simulink model "lqr_nao_linear_simulink"  (R2022a)
settings: Solver=VariableStepAuto  StartTime=0  StopTime=200  RelTol=1e-3
values from neighbouring files (symbols this model uses):
  A = [ 0 1 0  0 ... (first row only)    [ball_and_beam_pfc.m]
  amplitude_entrada = 1    [ball_and_beam_pfc.m]
  B = [0 ... (first row only)    [ball_and_beam_pfc.m]
  bool_degrau = 1    [ball_and_beam_pfc.m]
  C = [0 0 1 0]    [ball_and_beam_pfc.m]
  g = 9.8    [ball_and_beam_pfc.m]    (also in nonlinear_ball_and_beam.m)
  Jv = (1/2) * mv * L^2    (= 0.058703125)    [ball_and_beam_pfc.m]    (also in nonlinear_ball_and_beam.m)
  k_seguimento_lqr = K_nulo(1:4)    [ball_and_beam_pfc.m]
  ki_seguimento_lqr = K_nulo(5)    [ball_and_beam_pfc.m]
  L = 0.425    [ball_and_beam_pfc.m]    (also in nonlinear_ball_and_beam.m)
  L_observador = inv(T)*Lchp    [ball_and_beam_pfc.m]
  mb = 0.064    [ball_and_beam_pfc.m]    (also in nonlinear_ball_and_beam.m)
  mv = 0.65    [ball_and_beam_pfc.m]    (also in nonlinear_ball_and_beam.m)
libraries: mpclib x1
settings Model: Creator=Notebook_Artur  LastModifiedBy=Notebook_Artur

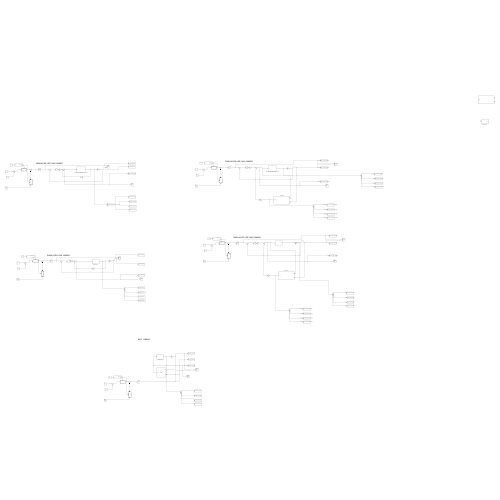
[thumbnail: Simulink's stored preview of the top-level diagram]
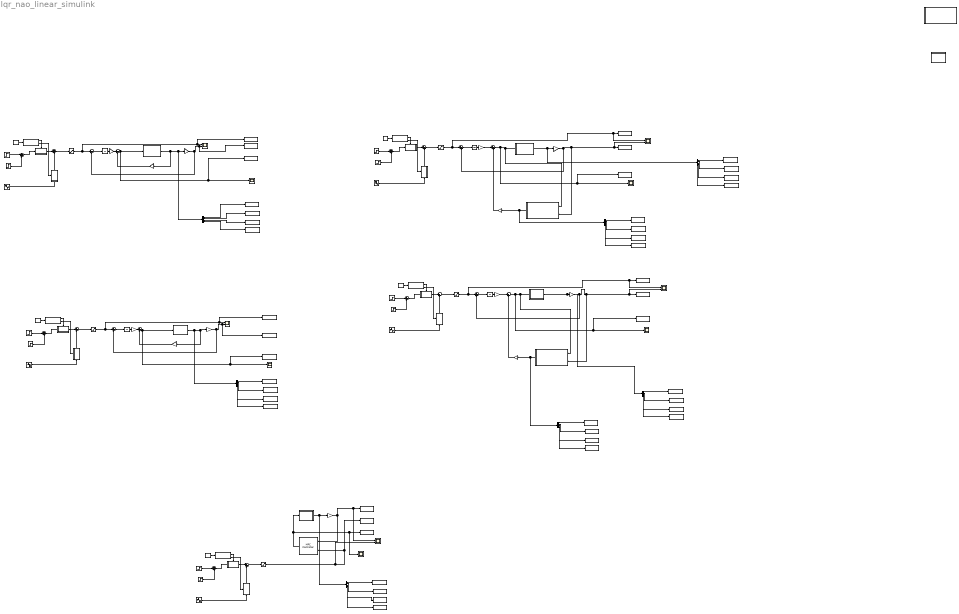
== system lqr_nao_linear_simulink ==
  note: SIMULAÇÃO LQR NAO LINEAR ENTRADA NORMAL
  note: SIMULAÇÃO LQR LINEAR ENTRADA NORMAL
  note: SIMULAÇÃO LQR NAO LINEAR ENTRADA NORMAL
  note: SIMULAÇÃO LQR NAO LINEAR ENTRADA NORMAL
  note: MPC LINEAR
  Constant{1..5} (5 alike) : Constant  Value=bool_degrau
  Demux{,1..6} (7 alike) : Demux
  Gain{1,4,7,29} (4 alike) : Gain  Gain=k_seguimento_lqr  Multiplication=Matrix(K*u)
  Gain{2,5,8,30,54} (5 alike) : Gain  Gain=C  Multiplication=Matrix(K*u)
  Gain{3,6,9,31} (4 alike) : Gain  Gain=ki_seguimento_lqr
  If{,1..4} (5 alike) : If  IfExpression=u1 == 1
  If Action Subsystem1 : Subsystem  TreatAsAtomicUnit=on
  If Action Subsystem10 : Subsystem  TreatAsAtomicUnit=on
  If Action Subsystem2 : Subsystem  TreatAsAtomicUnit=on
  If Action Subsystem3 : Subsystem  TreatAsAtomicUnit=on
  If Action Subsystem4 : Subsystem  TreatAsAtomicUnit=on
  If Action Subsystem5 : Subsystem  TreatAsAtomicUnit=on
  If Action Subsystem6 : Subsystem  TreatAsAtomicUnit=on
  If Action Subsystem7 : Subsystem  TreatAsAtomicUnit=on
  If Action Subsystem8 : Subsystem  TreatAsAtomicUnit=on
  If Action Subsystem9 : Subsystem  TreatAsAtomicUnit=on
  Integrator{1..3,5} (4 alike) : Integrator
  MPC Controller1 : mpclib/MPC Controller  SCDEnableBlockLinearizationSpecification=on  mpcobj=mpc1  is_multiple=0  enable_value=0  return_u0=off  updateMPCinCallerWorkspace=on  md_inport=off  mv_inport=off  uref_inport=off  return_cost=off  return_mvseq=off  return_qpstatus=off  return_xseq=off  return_state=off  return_ovseq=off  state_inport=off  umin_inport=off  umax_inport=off  ymin_inport=off  ymax_inport=off  cc_inport=off  ywt_inport=off  uwt_inport=off  duwt_inport=off  rhoeps_inport=off  pm_inport=off  MaximumP=10  HorizonChoice=FixedHorizon  n_ts=0.1  n_p=10  n_mv=1  n_md=0  n_ud=0  n_mo=1  n_uo=0  BlockDataType=double  SampleTimeInherited=off  switch_inport=off
  Modelo Linear : Subsystem
  Modelo Linear1 : Subsystem
  Modelo Linear2 : Subsystem
  Modelo Linear3 : Subsystem
  Modelo ball and beam nao linear - Final : Subsystem
  Modelo ball and beam nao linear - Final1 : Subsystem
  Observador1 : Subsystem
  Observador2 : Subsystem
  Observador3 : Subsystem
  Saturation{,1..4} (5 alike) : Saturate  UpperLimit=L/2  LowerLimit=-L/2
  Scope{,2..3,5,8} (5 alike) : Scope
  Scope{1,4,6..7,13} (5 alike) : Scope  NumInputPorts=2
  Sine Wave{1..5} (5 alike) : Sin  Amplitude=amplitude_entrada  Frequency=0.1  SampleTime=0
  Step{1,3,5..6,8} (5 alike) : Step  After=amplitude_entrada  SampleTime=0
  Step{2,4,7,9..10} (5 alike) : Step  Time=100  After=-2*amplitude_entrada  SampleTime=0
  Sum{,1,4..5,8..9,12..14,20} (10 alike) : Sum  Inputs=|++
  Sum{2..3,6..7,10..11,15..16} (8 alike) : Sum  Inputs=|+-
  To Workspace : ToWorkspace  VariableName=y_output_nao_linear  SaveFormat=Timeseries  SampleTime=-1
  To Workspace1 : ToWorkspace  VariableName=u_output_nao_linear  SaveFormat=Timeseries  SampleTime=-1
  To Workspace10 : ToWorkspace  VariableName=y_output_nao_linear_observador  SaveFormat=Timeseries  SampleTime=-1
  To Workspace11 : ToWorkspace  VariableName=u_output_nao_linear_observador  SaveFormat=Timeseries  SampleTime=-1
  To Workspace12 : ToWorkspace  VariableName=acao_controle_nao_linear_observador  SaveFormat=Timeseries  SampleTime=-1
  To Workspace13 : ToWorkspace  VariableName=estados_nao_linear_estimados_observador2  SaveFormat=Timeseries  SampleTime=-1
  To Workspace14 : ToWorkspace  VariableName=estados_linear1  SaveFormat=Timeseries  SampleTime=-1
  To Workspace15 : ToWorkspace  VariableName=estados_linear_observador1  SaveFormat=Timeseries  SampleTime=-1
  To Workspace16 : ToWorkspace  VariableName=estados_linear2  SaveFormat=Timeseries  SampleTime=-1
  To Workspace17 : ToWorkspace  VariableName=estados_linear3  SaveFormat=Timeseries  SampleTime=-1
  To Workspace18 : ToWorkspace  VariableName=estados_linear4  SaveFormat=Timeseries  SampleTime=-1
  To Workspace19 : ToWorkspace  VariableName=estados_nao_linear1  SaveFormat=Timeseries  SampleTime=-1
  To Workspace2 : ToWorkspace  VariableName=y_output_linear  SaveFormat=Timeseries  SampleTime=-1
  To Workspace20 : ToWorkspace  VariableName=estados_nao_linear2  SaveFormat=Timeseries  SampleTime=-1
  To Workspace21 : ToWorkspace  VariableName=estados_nao_linear3  SaveFormat=Timeseries  SampleTime=-1
  To Workspace22 : ToWorkspace  VariableName=estados_nao_linear4  SaveFormat=Timeseries  SampleTime=-1
  To Workspace23 : ToWorkspace  VariableName=estados_linear_observador2  SaveFormat=Timeseries  SampleTime=-1
  To Workspace24 : ToWorkspace  VariableName=estados_linear_observador3  SaveFormat=Timeseries  SampleTime=-1
  To Workspace25 : ToWorkspace  VariableName=estados_linear_observador4  SaveFormat=Timeseries  SampleTime=-1
  To Workspace26 : ToWorkspace  VariableName=estados_linear_estimados_observador1  SaveFormat=Timeseries  SampleTime=-1
  To Workspace27 : ToWorkspace  VariableName=estados_linear_estimados_observador2  SaveFormat=Timeseries  SampleTime=-1
  To Workspace28 : ToWorkspace  VariableName=estados_linear_estimados_observador3  SaveFormat=Timeseries  SampleTime=-1
  To Workspace29 : ToWorkspace  VariableName=estados_linear_estimados_observador4  SaveFormat=Timeseries  SampleTime=-1
  To Workspace3 : ToWorkspace  VariableName=u_output_linear  SaveFormat=Timeseries  SampleTime=-1
  To Workspace30 : ToWorkspace  VariableName=estados_nao_linear_estimados_observador3  SaveFormat=Timeseries  SampleTime=-1
  To Workspace31 : ToWorkspace  VariableName=estados_nao_linear_estimados_observador4  SaveFormat=Timeseries  SampleTime=-1
  To Workspace32 : ToWorkspace  VariableName=estados_nao_linear_observador1  SaveFormat=Timeseries  SampleTime=-1
  To Workspace33 : ToWorkspace  VariableName=estados_nao_linear_observador2  SaveFormat=Timeseries  SampleTime=-1
  To Workspace34 : ToWorkspace  VariableName=estados_nao_linear_observador3  SaveFormat=Timeseries  SampleTime=-1
  To Workspace35 : ToWorkspace  VariableName=estados_nao_linear_observador4  SaveFormat=Timeseries  SampleTime=-1
  To Workspace36 : ToWorkspace  VariableName=estados_mpc_linear1  SaveFormat=Timeseries  SampleTime=-1
  To Workspace37 : ToWorkspace  VariableName=estados_mpc_linear2  SaveFormat=Timeseries  SampleTime=-1
  To Workspace38 : ToWorkspace  VariableName=estados_mpc_linear3  SaveFormat=Timeseries  SampleTime=-1
  To Workspace39 : ToWorkspace  VariableName=estados_mpc_linear4  SaveFormat=Timeseries  SampleTime=-1
  To Workspace4 : ToWorkspace  VariableName=acao_controle_linear  SaveFormat=Timeseries  SampleTime=-1
  To Workspace40 : ToWorkspace  VariableName=y_output_mpc_linear  SaveFormat=Timeseries  SampleTime=-1
  To Workspace41 : ToWorkspace  VariableName=acao_controle_mpc_linear  SaveFormat=Timeseries  SampleTime=-1
  To Workspace42 : ToWorkspace  VariableName=u_output_mpc_linear  SaveFormat=Timeseries  SampleTime=-1
  To Workspace5 : ToWorkspace  VariableName=acao_controle_nao_linear  SaveFormat=Timeseries  SampleTime=-1
  To Workspace6 : ToWorkspace  VariableName=y_output_linear_observador  SaveFormat=Timeseries  SampleTime=-1
  To Workspace7 : ToWorkspace  VariableName=u_output_linear_observador  SaveFormat=Timeseries  SampleTime=-1
  To Workspace8 : ToWorkspace  VariableName=acao_controle_linear_observador  SaveFormat=Timeseries  SampleTime=-1
  To Workspace9 : ToWorkspace  VariableName=estados_nao_linear_estimados_observador1  SaveFormat=Timeseries  SampleTime=-1
  wires:
  Sum16/1 -> Integrator5/1
  Gain30/1 -> Sum16/2, To Workspace/1, Scope13/2
  Step9/1 -> Sum20/2
  Gain29/1 -> Sum15/2
  Step6/1 -> Sum20/1
  Gain31/1 -> Sum15/1
  Integrator5/1 -> Gain31/1
  Saturation/1 -> To Workspace1/1, Scope13/1, Sum16/1
  Sine Wave1/1 -> If Action Subsystem1/1(In1)
  If Action Subsystem1/1(Out1) -> Sum/2
  Sum20/1 -> If Action Subsystem2/1(In1)
  If Action Subsystem2/1(Out1) -> Sum/1
  Sum/1 -> Saturation/1
  Constant2/1 -> If/1
  If/1 -> If Action Subsystem2/Action
  If/2 -> If Action Subsystem1/Action
  Sum15/1 -> Modelo ball and beam nao linear - Final/1(In1), To Workspace5/1, Scope2/1
  If1/1 -> If Action Subsystem4/Action
  If Action Subsystem3/1(Out1) -> Sum1/2
  Sum1/1 -> Saturation1/1
  If Action Subsystem4/1(Out1) -> Sum1/1
  If1/2 -> If Action Subsystem3/Action
  Integrator1/1 -> Gain3/1
  Gain3/1 -> Sum2/1
  Step1/1 -> Sum4/1
  Sine Wave2/1 -> If Action Subsystem3/1(In1)
  Sum2/1 -> Modelo Linear1/1(Input), To Workspace4/1, Scope3/1
  Gain1/1 -> Sum2/2
  Saturation1/1 -> To Workspace3/1, Scope1/1, Sum3/1
  Sum3/1 -> Integrator1/1
  Sum4/1 -> If Action Subsystem4/1(In1)
  Gain2/1 -> Sum3/2, To Workspace2/1, Scope1/2
  Step2/1 -> Sum4/2
  Constant1/1 -> If1/1
  Constant3/1 -> If2/1
  Modelo Linear2/1(Output) -> Demux2/1, Gain5/1
  If2/1 -> If Action Subsystem6/Action
  Gain4/1 -> Sum6/2
  Step4/1 -> Sum8/2
  Sum6/1 -> To Workspace8/1, Scope5/1, Observador1/1(ref), Modelo Linear2/1(Input)
  Sum7/1 -> Integrator2/1
  Gain5/1 -> Sum7/2, Scope4/2, To Workspace6/1, Observador1/2(y)
  Saturation2/1 -> To Workspace7/1, Scope4/1, Sum7/1
  Step3/1 -> Sum8/1
  Gain6/1 -> Sum6/1
  If Action Subsystem6/1(Out1) -> Sum5/1
  Sum5/1 -> Saturation2/1
  Integrator2/1 -> Gain6/1
  If2/2 -> If Action Subsystem5/Action
  Sine Wave3/1 -> If Action Subsystem5/1(In1)
  Sum8/1 -> If Action Subsystem6/1(In1)
  If Action Subsystem5/1(Out1) -> Sum5/2
  Observador1/1(x_chp) -> Demux3/1, Gain4/1
  If Action Subsystem7/1(Out1) -> Sum9/2
  If Action Subsystem8/1(Out1) -> Sum9/1
  If3/2 -> If Action Subsystem7/Action
  Gain9/1 -> Sum10/1
  Step5/1 -> Sum12/1
  Sine Wave4/1 -> If Action Subsystem7/1(In1)
  Integrator3/1 -> Gain9/1
  Sum12/1 -> If Action Subsystem8/1(In1)
  Saturation3/1 -> To Workspace11/1, Scope7/1, Sum11/1
  Sum9/1 -> Saturation3/1
  Gain8/1 -> Scope7/2, To Workspace10/1, Observador3/2(y), Sum11/2
  Constant4/1 -> If3/1
  Gain7/1 -> Sum10/2
  Sum10/1 -> To Workspace12/1, Scope8/1, Observador3/1(ref), Modelo ball and beam nao linear - Final1/1(In1)
  If3/1 -> If Action Subsystem8/Action
  Observador3/1(x_chp) -> Demux4/1, Gain7/1
  Step7/1 -> Sum12/2
  Sum11/1 -> Integrator3/1
  Modelo ball and beam nao linear - Final1/1(Out1) -> Demux5/1, Gain8/1
  Modelo Linear1/1(Output) -> Demux/1, Gain2/1, Gain1/1
  Modelo ball and beam nao linear - Final/1(Out1) -> Demux1/1, Gain30/1, Gain29/1
  Demux/1 -> To Workspace14/1
  Demux/2 -> To Workspace16/1
  Demux/3 -> To Workspace17/1
  Demux/4 -> To Workspace18/1
  Demux1/3 -> To Workspace21/1
  Demux1/4 -> To Workspace22/1
  Demux1/2 -> To Workspace20/1
  Demux1/1 -> To Workspace19/1
  Demux2/3 -> To Workspace24/1
  Demux2/4 -> To Workspace25/1
  Demux2/2 -> To Workspace23/1
  Demux2/1 -> To Workspace15/1
  Demux3/1 -> To Workspace26/1
  Demux3/4 -> To Workspace29/1
  Demux3/3 -> To Workspace28/1
  Demux3/2 -> To Workspace27/1
  Demux4/1 -> To Workspace9/1
  Demux4/4 -> To Workspace31/1
  Demux4/2 -> To Workspace13/1
  Demux4/3 -> To Workspace30/1
  Demux5/1 -> To Workspace32/1
  Demux5/4 -> To Workspace35/1
  Demux5/3 -> To Workspace34/1
  Demux5/2 -> To Workspace33/1
  Sine Wave5/1 -> If Action Subsystem9/1(In1)
  Sum14/1 -> If Action Subsystem10/1(In1)
  If4/2 -> If Action Subsystem9/Action
  Sum13/1 -> Saturation4/1
  If Action Subsystem10/1(Out1) -> Sum13/1
  Step8/1 -> Sum14/1
  If Action Subsystem9/1(Out1) -> Sum13/2
  Step10/1 -> Sum14/2
  Constant5/1 -> If4/1
  If4/1 -> If Action Subsystem10/Action
  MPC Controller1/1 -> Modelo Linear3/1(Input), Scope/1, To Workspace41/1
  Gain54/1 -> Scope6/1, To Workspace40/1, MPC Controller1/1
  Saturation4/1 -> Scope6/2, MPC Controller1/2, To Workspace42/1
  Demux6/4 -> To Workspace39/1
  Demux6/1 -> To Workspace36/1
  Demux6/3 -> To Workspace38/1
  Demux6/2 -> To Workspace37/1
  Modelo Linear3/1(Output) -> Demux6/1, Gain54/1

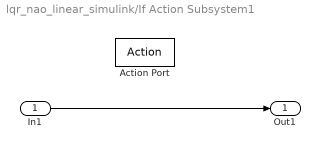
== system lqr_nao_linear_simulink/If Action Subsystem1 ==
  In1 : Inport
  Action Port : ActionPort  ActionPortLabel=else
  Out1 : Outport
  wires:
  In1/1 -> Out1/1

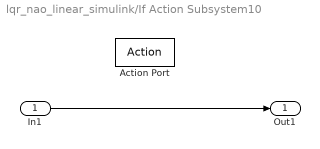
== system lqr_nao_linear_simulink/If Action Subsystem10 ==
  In1 : Inport
  Action Port : ActionPort  ActionPortLabel=if(u1 == 1)
  Out1 : Outport
  wires:
  In1/1 -> Out1/1

== system lqr_nao_linear_simulink/If Action Subsystem2 ==
  In1 : Inport
  Action Port : ActionPort  ActionPortLabel=if(u1 == 1)
  Out1 : Outport
  wires:
  In1/1 -> Out1/1

== system lqr_nao_linear_simulink/If Action Subsystem3 ==
  In1 : Inport
  Action Port : ActionPort  ActionPortLabel=else
  Out1 : Outport
  wires:
  In1/1 -> Out1/1

== system lqr_nao_linear_simulink/If Action Subsystem4 ==
  In1 : Inport
  Action Port : ActionPort  ActionPortLabel=if(u1 == 1)
  Out1 : Outport
  wires:
  In1/1 -> Out1/1

== system lqr_nao_linear_simulink/If Action Subsystem5 ==
  In1 : Inport
  Action Port : ActionPort  ActionPortLabel=else
  Out1 : Outport
  wires:
  In1/1 -> Out1/1

== system lqr_nao_linear_simulink/If Action Subsystem6 ==
  In1 : Inport
  Action Port : ActionPort  ActionPortLabel=if(u1 == 1)
  Out1 : Outport
  wires:
  In1/1 -> Out1/1

== system lqr_nao_linear_simulink/If Action Subsystem7 ==
  In1 : Inport
  Action Port : ActionPort  ActionPortLabel=else
  Out1 : Outport
  wires:
  In1/1 -> Out1/1

== system lqr_nao_linear_simulink/If Action Subsystem8 ==
  In1 : Inport
  Action Port : ActionPort  ActionPortLabel=if(u1 == 1)
  Out1 : Outport
  wires:
  In1/1 -> Out1/1

== system lqr_nao_linear_simulink/If Action Subsystem9 ==
  In1 : Inport
  Action Port : ActionPort  ActionPortLabel=else
  Out1 : Outport
  wires:
  In1/1 -> Out1/1

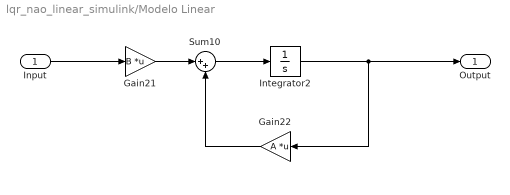
== system lqr_nao_linear_simulink/Modelo Linear ==
  Input : Inport
  Gain21 : Gain  Gain=B  Multiplication=Matrix(K*u)
  Gain22 : Gain  Gain=A  Multiplication=Matrix(K*u)
  Integrator2 : Integrator
  Sum10 : Sum  Inputs=|++
  Output : Outport
  wires:
  Input/1 -> Gain21/1
  Gain22/1 -> Sum10/2
  Integrator2/1 -> Output/1, Gain22/1
  Gain21/1 -> Sum10/1
  Sum10/1 -> Integrator2/1

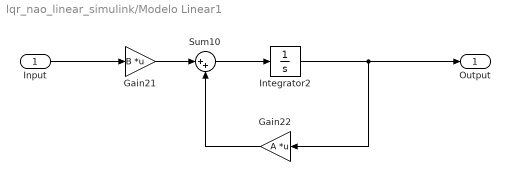
== system lqr_nao_linear_simulink/Modelo Linear1 ==
  Input : Inport
  Gain21 : Gain  Gain=B  Multiplication=Matrix(K*u)
  Gain22 : Gain  Gain=A  Multiplication=Matrix(K*u)
  Integrator2 : Integrator
  Sum10 : Sum  Inputs=|++
  Output : Outport
  wires:
  Input/1 -> Gain21/1
  Gain22/1 -> Sum10/2
  Integrator2/1 -> Output/1, Gain22/1
  Gain21/1 -> Sum10/1
  Sum10/1 -> Integrator2/1

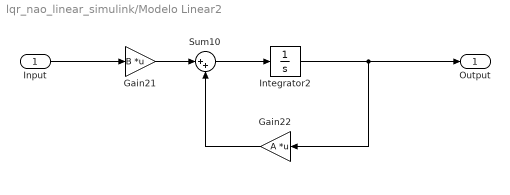
== system lqr_nao_linear_simulink/Modelo Linear2 ==
  Input : Inport
  Gain21 : Gain  Gain=B  Multiplication=Matrix(K*u)
  Gain22 : Gain  Gain=A  Multiplication=Matrix(K*u)
  Integrator2 : Integrator
  Sum10 : Sum  Inputs=|++
  Output : Outport
  wires:
  Input/1 -> Gain21/1
  Gain22/1 -> Sum10/2
  Integrator2/1 -> Output/1, Gain22/1
  Gain21/1 -> Sum10/1
  Sum10/1 -> Integrator2/1

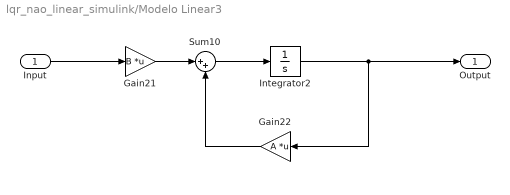
== system lqr_nao_linear_simulink/Modelo Linear3 ==
  Input : Inport
  Gain21 : Gain  Gain=B  Multiplication=Matrix(K*u)
  Gain22 : Gain  Gain=A  Multiplication=Matrix(K*u)
  Integrator2 : Integrator
  Sum10 : Sum  Inputs=|++
  Output : Outport
  wires:
  Input/1 -> Gain21/1
  Gain22/1 -> Sum10/2
  Integrator2/1 -> Output/1, Gain22/1
  Gain21/1 -> Sum10/1
  Sum10/1 -> Integrator2/1

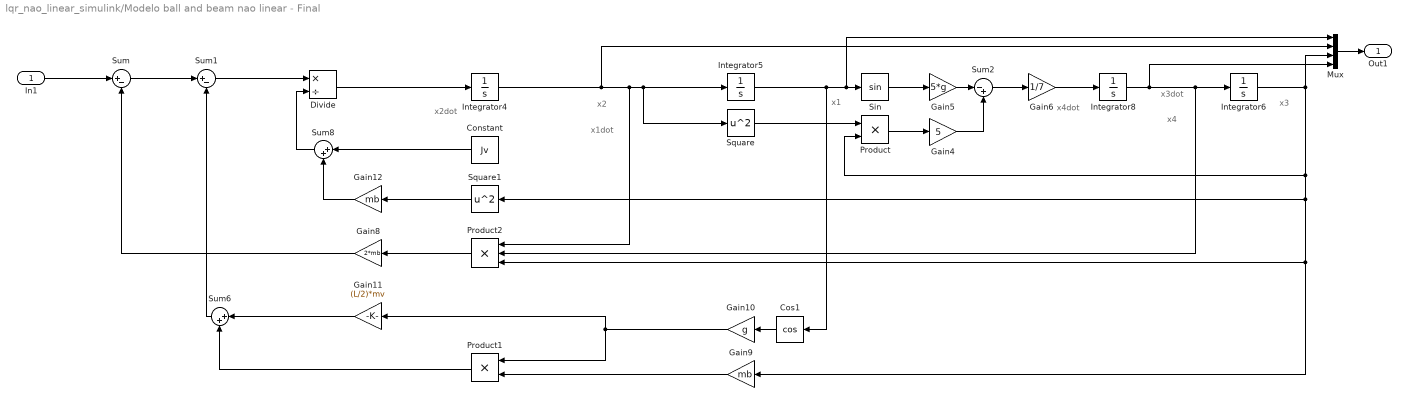
== system lqr_nao_linear_simulink/Modelo ball and beam nao linear - Final ==
  note: x3
  note: x3dot
  note: x4
  note: x4dot
  note: x1
  note: x1dot
  note: x2dot
  note: x2
  In1 : Inport
  Constant : Constant  Value=Jv
  Cos1 : Trigonometry  Operator=cos
  Divide : Product  Inputs=*/
  Gain10 : Gain  Gain=g
  Gain11 : Gain  Gain=(L/2)*mv
  Gain12 : Gain  Gain=mb
  Gain4 : Gain  Gain=5
  Gain5 : Gain  Gain=5*g
  Gain6 : Gain  Gain=1/7
  Gain8 : Gain  Gain=2*mb
  Gain9 : Gain  Gain=mb
  Integrator{4..6,8} (4 alike) : Integrator
  Mux : Mux
  Product : Product
  Product1 : Product
  Product2 : Product  Inputs=3
  Sin : Trigonometry
  Square : Math  Operator=square
  Square1 : Math  Operator=square
  Sum : Sum  Inputs=|+-
  Sum1 : Sum  Inputs=|+-
  Sum2 : Sum  Inputs=|-+
  Sum6 : Sum  Inputs=|++
  Sum8 : Sum  Inputs=|++
  Out1 : Outport
  wires:
  Integrator8/1 -> Mux/4, Product2/2, Integrator6/1
  Integrator5/1 -> Cos1/1, Mux/1, Sin/1
  Sum6/1 -> Sum1/2
  Sum2/1 -> Gain6/1
  Gain10/1 -> Product1/1, Gain11/1
  Square/1 -> Product/1
  Integrator6/1 -> Mux/3, Gain9/1, Product2/3, Square1/1, Product/2
  Gain11/1 -> Sum6/1
  Gain12/1 -> Sum8/2
  Gain6/1 -> Integrator8/1
  Gain4/1 -> Sum2/2
  Gain9/1 -> Product1/2
  Cos1/1 -> Gain10/1
  Divide/1 -> Integrator4/1
  Product2/1 -> Gain8/1
  Product/1 -> Gain4/1
  Square1/1 -> Gain12/1
  Sum8/1 -> Divide/2
  Product1/1 -> Sum6/2
  Constant/1 -> Sum8/1
  Mux/1 -> Out1/1
  Gain5/1 -> Sum2/1
  Sin/1 -> Gain5/1
  Gain8/1 -> Sum/2
  Sum1/1 -> Divide/1
  Sum/1 -> Sum1/1
  Integrator4/1 -> Mux/2, Product2/1, Square/1, Integrator5/1
  In1/1 -> Sum/1

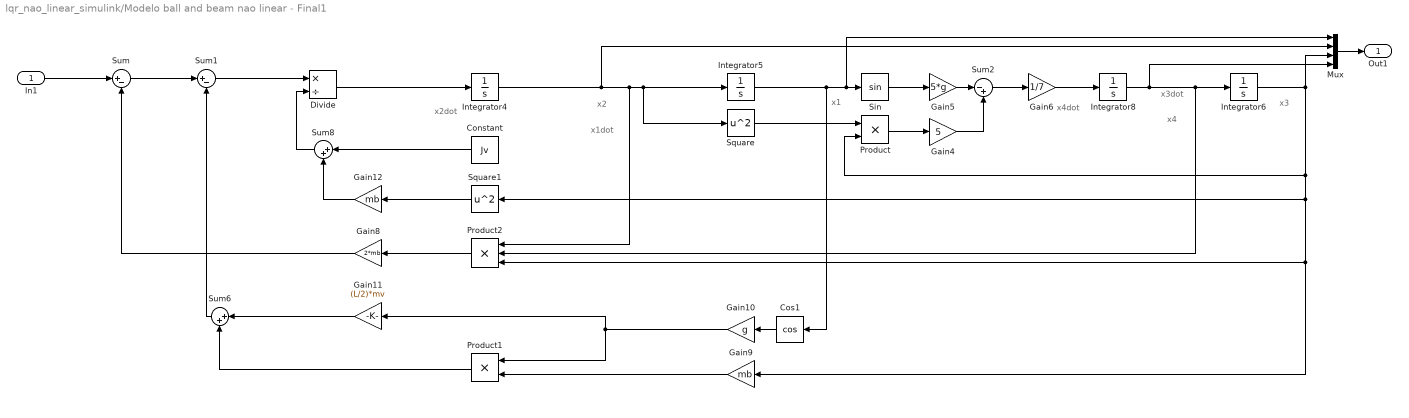
== system lqr_nao_linear_simulink/Modelo ball and beam nao linear - Final1 ==
  note: x3
  note: x3dot
  note: x4
  note: x4dot
  note: x1
  note: x1dot
  note: x2dot
  note: x2
  In1 : Inport
  Constant : Constant  Value=Jv
  Cos1 : Trigonometry  Operator=cos
  Divide : Product  Inputs=*/
  Gain10 : Gain  Gain=g
  Gain11 : Gain  Gain=(L/2)*mv
  Gain12 : Gain  Gain=mb
  Gain4 : Gain  Gain=5
  Gain5 : Gain  Gain=5*g
  Gain6 : Gain  Gain=1/7
  Gain8 : Gain  Gain=2*mb
  Gain9 : Gain  Gain=mb
  Integrator{4..6,8} (4 alike) : Integrator
  Mux : Mux
  Product : Product
  Product1 : Product
  Product2 : Product  Inputs=3
  Sin : Trigonometry
  Square : Math  Operator=square
  Square1 : Math  Operator=square
  Sum : Sum  Inputs=|+-
  Sum1 : Sum  Inputs=|+-
  Sum2 : Sum  Inputs=|-+
  Sum6 : Sum  Inputs=|++
  Sum8 : Sum  Inputs=|++
  Out1 : Outport
  wires:
  Integrator8/1 -> Mux/4, Product2/2, Integrator6/1
  Integrator5/1 -> Cos1/1, Mux/1, Sin/1
  Sum6/1 -> Sum1/2
  Sum2/1 -> Gain6/1
  Gain10/1 -> Product1/1, Gain11/1
  Square/1 -> Product/1
  Integrator6/1 -> Mux/3, Gain9/1, Product2/3, Square1/1, Product/2
  Gain11/1 -> Sum6/1
  Gain12/1 -> Sum8/2
  Gain6/1 -> Integrator8/1
  Gain4/1 -> Sum2/2
  Gain9/1 -> Product1/2
  Cos1/1 -> Gain10/1
  Divide/1 -> Integrator4/1
  Product2/1 -> Gain8/1
  Product/1 -> Gain4/1
  Square1/1 -> Gain12/1
  Sum8/1 -> Divide/2
  Product1/1 -> Sum6/2
  Constant/1 -> Sum8/1
  Mux/1 -> Out1/1
  Gain5/1 -> Sum2/1
  Sin/1 -> Gain5/1
  Gain8/1 -> Sum/2
  Sum1/1 -> Divide/1
  Sum/1 -> Sum1/1
  Integrator4/1 -> Mux/2, Product2/1, Square/1, Integrator5/1
  In1/1 -> Sum/1

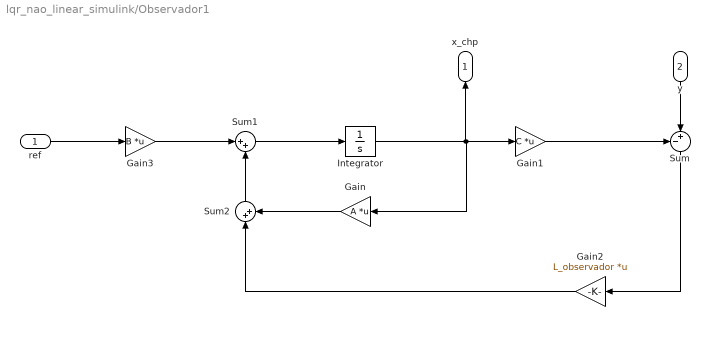
== system lqr_nao_linear_simulink/Observador1 ==
  ref : Inport
  y : Inport  Port=2
  Gain : Gain  Gain=A  Multiplication=Matrix(K*u)
  Gain1 : Gain  Gain=C  Multiplication=Matrix(K*u)
  Gain2 : Gain  Gain=L_observador  Multiplication=Matrix(K*u)
  Gain3 : Gain  Gain=B  Multiplication=Matrix(K*u)
  Integrator : Integrator
  Sum : Sum  Inputs=-+|
  Sum1 : Sum  Inputs=|++
  Sum2 : Sum  Inputs=|++
  x_chp : Outport
  wires:
  Integrator/1 -> x_chp/1, Gain1/1, Gain/1
  Sum/1 -> Gain2/1
  Gain1/1 -> Sum/1
  Gain/1 -> Sum2/2
  y/1 -> Sum/2
  Sum2/1 -> Sum1/2
  Gain2/1 -> Sum2/1
  Sum1/1 -> Integrator/1
  ref/1 -> Gain3/1
  Gain3/1 -> Sum1/1

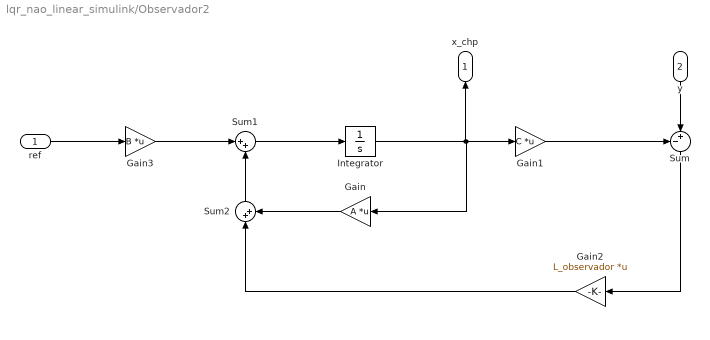
== system lqr_nao_linear_simulink/Observador2 ==
  ref : Inport
  y : Inport  Port=2
  Gain : Gain  Gain=A  Multiplication=Matrix(K*u)
  Gain1 : Gain  Gain=C  Multiplication=Matrix(K*u)
  Gain2 : Gain  Gain=L_observador  Multiplication=Matrix(K*u)
  Gain3 : Gain  Gain=B  Multiplication=Matrix(K*u)
  Integrator : Integrator
  Sum : Sum  Inputs=-+|
  Sum1 : Sum  Inputs=|++
  Sum2 : Sum  Inputs=|++
  x_chp : Outport
  wires:
  Integrator/1 -> x_chp/1, Gain1/1, Gain/1
  Sum/1 -> Gain2/1
  Gain1/1 -> Sum/1
  Gain/1 -> Sum2/2
  y/1 -> Sum/2
  Sum2/1 -> Sum1/2
  Gain2/1 -> Sum2/1
  Sum1/1 -> Integrator/1
  ref/1 -> Gain3/1
  Gain3/1 -> Sum1/1

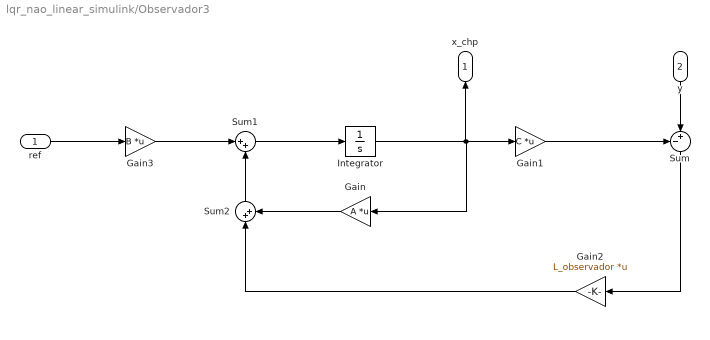
== system lqr_nao_linear_simulink/Observador3 ==
  ref : Inport
  y : Inport  Port=2
  Gain : Gain  Gain=A  Multiplication=Matrix(K*u)
  Gain1 : Gain  Gain=C  Multiplication=Matrix(K*u)
  Gain2 : Gain  Gain=L_observador  Multiplication=Matrix(K*u)
  Gain3 : Gain  Gain=B  Multiplication=Matrix(K*u)
  Integrator : Integrator
  Sum : Sum  Inputs=-+|
  Sum1 : Sum  Inputs=|++
  Sum2 : Sum  Inputs=|++
  x_chp : Outport
  wires:
  Integrator/1 -> x_chp/1, Gain1/1, Gain/1
  Sum/1 -> Gain2/1
  Gain1/1 -> Sum/1
  Gain/1 -> Sum2/2
  y/1 -> Sum/2
  Sum2/1 -> Sum1/2
  Gain2/1 -> Sum2/1
  Sum1/1 -> Integrator/1
  ref/1 -> Gain3/1
  Gain3/1 -> Sum1/1
